simulink model "propeller_research"  (R2014b)
settings: Solver=ode45  StartTime=0.0  StopTime=10.0  RelTol=1e-3
settings Model: Creator=Vlad  LastModifiedBy=Vlad

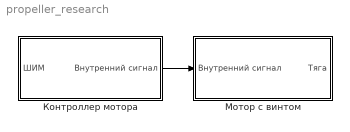
== system propeller_research ==
  "Контроллер мотора " : Subsystem  TreatAsAtomicUnit=on
  Мотор с винтом : Subsystem  TreatAsAtomicUnit=on
  wires:
  "Контроллер мотора "/1(Внутренний сигнал) -> Мотор с винтом/1("Внутренний сигнал ")

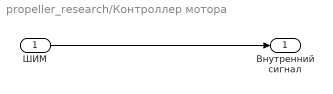
== system propeller_research/Контроллер мотора  ==
  ШИМ : Inport
  Внутренний сигнал : Outport
  wires:
  ШИМ/1 -> Внутренний сигнал/1

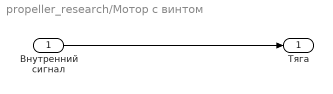
== system propeller_research/Мотор с винтом ==
  "Внутренний сигнал " : Inport
  "Тяга " : Outport
  wires:
  "Внутренний сигнал "/1 -> "Тяга "/1
